simulink model "SMO_simulink"  (R2023b)
settings: Solver=VariableStepAuto  StartTime=0.0  StopTime=10.0  RelTol=1e-3
settings Model: Creator=jjake  LastModifiedBy=jjake

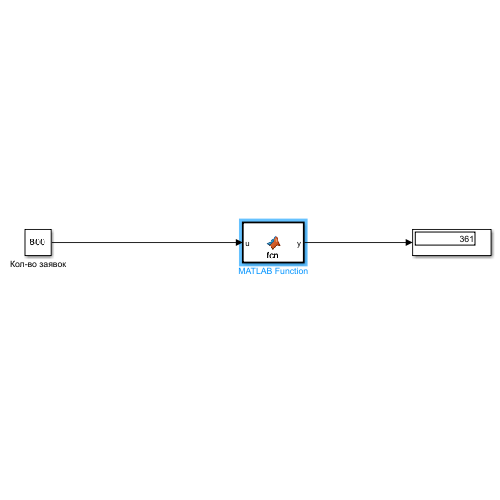
[thumbnail: Simulink's stored preview of the top-level diagram]
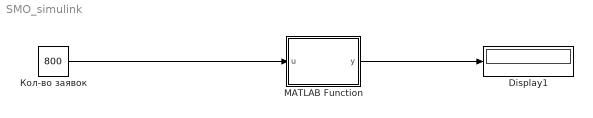
== system SMO_simulink ==
  Display1 : Display
  MATLAB Function : MATLAB Function  TreatAsAtomicUnit=on
  Кол-во заявок : Constant  Value=800
  wires:
  Кол-во заявок/1 -> MATLAB Function/1(u)
  MATLAB Function/1(y) -> Display1/1

== matlab function SMO_simulink/MATLAB Function ==
  data: u input; y output
function y = fcn(u)
   %define params
    lambda = 30;
    mu = 20;
    n = 6;
    m = 5;
    
    %compute mark chain params
    rho = lambda/mu;
    
    p0 = 1 / (sum(arrayfun(@(k) rho^k/factorial(k), 0:n-1)) + rho^n/factorial(n) * (1-rho^m)/(1-rho));
    
    P_otk = rho^(n+m)/(n^m*factorial(n)) * p0;
    
    Q = 1 - P_otk;
    
    A = lambda * Q;
    
    k_zan = A / mu;
    
    L_och = (rho^(n+1)/(n*factorial(n))) * (1 - (rho/n)^m * (m+1 - m*rho/n)) / (1 - rho/n)^2 * p0;
    
    T_och = L_och / lambda;
    
    L_sist = L_och + k_zan;
    
    T_sist = L_sist / lambda;
    
    result = zeros(1000, 1);

    for i = 1 : u
       r = rand();

        if r >= P_otk
            result(i) = 1;
        else
            result(i) = 0;
        end
    end

    y = sum(result);
end
